simulink library "ArbolFallosLIB__"  (Simulink 6.0)
settings Model: Creator=Luis  LastModifiedBy=Luis  CovMetricSettings=dwe  CovHtmlReporting=off  covSaveCumulativeToWorkspaceVar=off  CovSaveSingleToWorkspaceVar=off  CovExternalEMLEnable=on

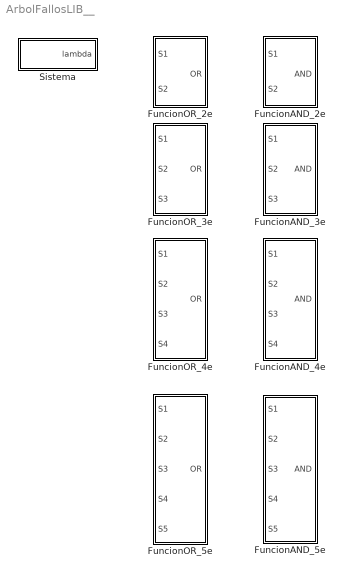
== system ArbolFallosLIB__ ==
  FuncionAND_2e : Subsystem
      mask Display:
      | port_label('input',1,'S_1','texmode','on');
      | port_label('input',2,'S_2','texmode','on');
      | port_label('output',1,'\lambda','texmode','on');
      | fprintf('AND');
  FuncionAND_3e : Subsystem
      mask Display:
      | port_label('input',1,'S_1','texmode','on');
      | port_label('input',2,'S_2','texmode','on');
      | port_label('input',3,'S_3','texmode','on');
      | port_label('output',1,'\lambda','texmode','on');
      | fprintf('AND');
  FuncionAND_4e : Subsystem
      mask Display:
      | port_label('input',1,'S_1','texmode','on');
      | port_label('input',2,'S_2','texmode','on');
      | port_label('input',3,'S_3','texmode','on');
      | port_label('input',4,'S_4','texmode','on');
      | port_label('output',1,'\lambda','texmode','on');
      | fprintf('AND');
  FuncionAND_5e : Subsystem
      mask Display:
      | port_label('input',1,'S_1','texmode','on');
      | port_label('input',2,'S_2','texmode','on');
      | port_label('input',3,'S_3','texmode','on');
      | port_label('input',4,'S_4','texmode','on');
      | port_label('input',5,'S_5','texmode','on');
      | port_label('output',1,'\lambda','texmode','on');
      | fprintf('AND');
  FuncionOR_2e : Subsystem
      mask Display:
      | port_label('input',1,'S_1','texmode','on');
      | port_label('input',2,'S_2','texmode','on');
      | port_label('output',1,'\lambda','texmode','on');
      | fprintf('OR');
  FuncionOR_3e : Subsystem
      mask Display:
      | port_label('input',1,'S_1','texmode','on');
      | port_label('input',2,'S_2','texmode','on');
      | port_label('input',3,'S_3','texmode','on');
      | port_label('output',1,'\lambda','texmode','on');
      | fprintf('OR');
  FuncionOR_4e : Subsystem
      mask Display:
      | port_label('input',1,'S_1','texmode','on');
      | port_label('input',2,'S_2','texmode','on');
      | port_label('input',3,'S_3','texmode','on');
      | port_label('input',4,'S_4','texmode','on');
      | port_label('output',1,'\lambda','texmode','on');
      | fprintf('OR');
  FuncionOR_5e : Subsystem
      mask Display:
      | port_label('input',1,'S_1','texmode','on');
      | port_label('input',2,'S_2','texmode','on');
      | port_label('input',3,'S_3','texmode','on');
      | port_label('input',4,'S_4','texmode','on');
      | port_label('input',5,'S_5','texmode','on');
      | port_label('output',1,'\lambda','texmode','on');
      | fprintf('OR');
  Sistema : Subsystem  mask{sistema='Sistema', lambda=1e-3}
      mask prompts: sistema "Nombre del sistema"; lambda "Probabilidad de fallo"
      mask Display:
      | fprintf('%s\n(%3.1e)',sistema,lambda);
      | port_label('output',1,'\lambda','texmode','on');

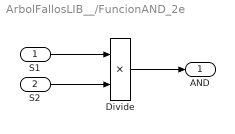
== system ArbolFallosLIB__/FuncionAND_2e ==
  S1 : Inport
  S2 : Inport  Port=2
  Divide : Product  Inputs=**
  AND : Outport
  wires:
  Divide/1 -> AND/1
  S1/1 -> Divide/1
  S2/1 -> Divide/2

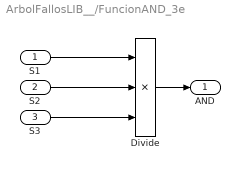
== system ArbolFallosLIB__/FuncionAND_3e ==
  S1 : Inport
  S2 : Inport  Port=2
  S3 : Inport  Port=3
  Divide : Product  Inputs=***
  AND : Outport
  wires:
  S1/1 -> Divide/1
  S2/1 -> Divide/2
  S3/1 -> Divide/3
  Divide/1 -> AND/1

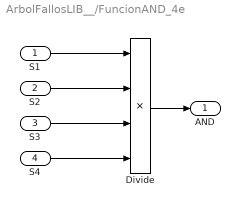
== system ArbolFallosLIB__/FuncionAND_4e ==
  S1 : Inport
  S2 : Inport  Port=2
  S3 : Inport  Port=3
  S4 : Inport  Port=4
  Divide : Product  Inputs=****
  AND : Outport
  wires:
  S1/1 -> Divide/1
  S2/1 -> Divide/2
  S3/1 -> Divide/3
  Divide/1 -> AND/1
  S4/1 -> Divide/4

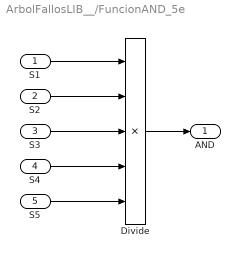
== system ArbolFallosLIB__/FuncionAND_5e ==
  S1 : Inport
  S2 : Inport  Port=2
  S3 : Inport  Port=3
  S4 : Inport  Port=4
  S5 : Inport  Port=5
  Divide : Product  Inputs=*****
  AND : Outport
  wires:
  S1/1 -> Divide/1
  S2/1 -> Divide/2
  S3/1 -> Divide/3
  Divide/1 -> AND/1
  S4/1 -> Divide/4
  S5/1 -> Divide/5

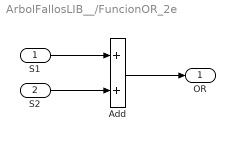
== system ArbolFallosLIB__/FuncionOR_2e ==
  S1 : Inport
  S2 : Inport  Port=2
  Add : Sum
  OR : Outport
  wires:
  Add/1 -> OR/1
  S1/1 -> Add/1
  S2/1 -> Add/2

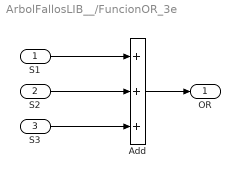
== system ArbolFallosLIB__/FuncionOR_3e ==
  S1 : Inport
  S2 : Inport  Port=2
  S3 : Inport  Port=3
  Add : Sum  Inputs=+++
  OR : Outport
  wires:
  S1/1 -> Add/1
  S2/1 -> Add/2
  S3/1 -> Add/3
  Add/1 -> OR/1

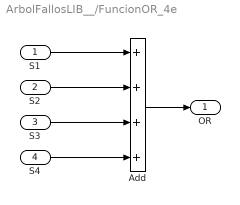
== system ArbolFallosLIB__/FuncionOR_4e ==
  S1 : Inport
  S2 : Inport  Port=2
  S3 : Inport  Port=3
  S4 : Inport  Port=4
  Add : Sum  Inputs=++++
  OR : Outport
  wires:
  S1/1 -> Add/1
  S2/1 -> Add/2
  S3/1 -> Add/3
  Add/1 -> OR/1
  S4/1 -> Add/4

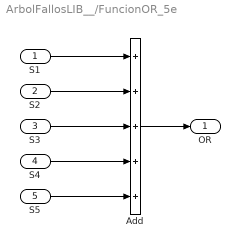
== system ArbolFallosLIB__/FuncionOR_5e ==
  S1 : Inport
  S2 : Inport  Port=2
  S3 : Inport  Port=3
  S4 : Inport  Port=4
  S5 : Inport  Port=5
  Add : Sum  Inputs=+++++
  OR : Outport
  wires:
  S1/1 -> Add/1
  S2/1 -> Add/2
  S3/1 -> Add/3
  Add/1 -> OR/1
  S4/1 -> Add/4
  S5/1 -> Add/5

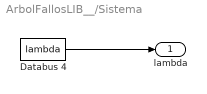
== system ArbolFallosLIB__/Sistema ==
  Databus 4 : Constant  Value=lambda
  lambda : Outport
  wires:
  Databus 4/1 -> lambda/1
